simulink model "model1"  (R2019b)
settings: Solver=VariableStepAuto  StartTime=0.0  StopTime=tSimulation  RelTol=1e-3
values from neighbouring files (symbols this model uses):
  a = 1    [param1a.m]    (also in param1b.m = 0.1)
  alpha2 = 3*a    (= 3)    [param1a.m]    (also in param1b.m = 0.3)
  dAmplitude = -1    [param1a.m]    (also in param1b.m)
  Gs = tf(1, den)    [param1a.m]    (also in param1b.m)
  K1 = (alpha1 - a)/b    (= 10)    [param1a.m]    (also in param1b.m = 5; param2.m = 5)
  K2 = alpha2/b    (= 30)    [param1a.m]    (also in param1b.m = 15; param2.m = 2.121)
  tDelay = 0.01    [param1a.m]    (also in param1b.m)
  tDelta = 0.001    [param1a.m]    (also in param1b.m)
  tDist = tSimulation/2    (= 15)    [param1a.m]    (also in param1b.m)
  umax = 999    [param1a.m]    (also in param1b.m = 34)
  umin = -999    [param1a.m]    (also in param1b.m = -10.2)
settings Model: Creator=adityaaaap  LastModifiedBy=adityaaaap

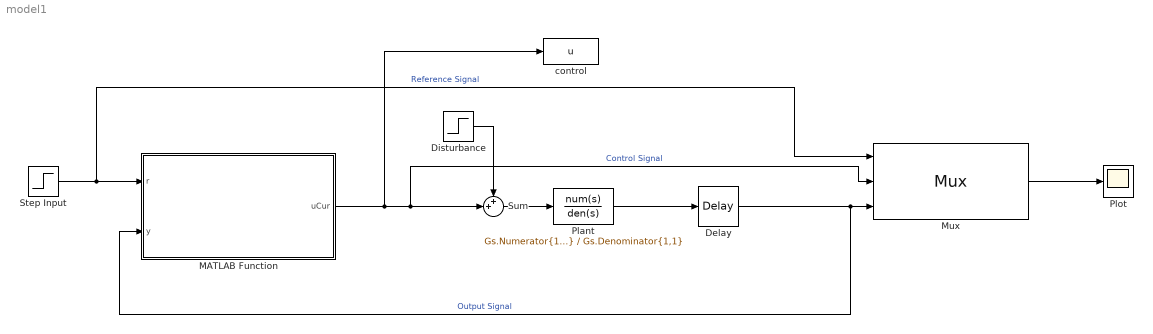
== system model1 ==
  Delay : TransportDelay  DelayTime=tDelay
  Disturbance : Step  Time=tDist  After=dAmplitude  SampleTime=0
  MATLAB Function : MATLAB Function  TreatAsAtomicUnit=on
  Mux : Mux  Inputs=3
      settings: DisplayOption=signals
  Plant : TransferFcn  Numerator=Gs.Numerator{1,1}  Denominator=Gs.Denominator{1,1}
  Plot : Scope
  Step Input : Step  Time=0  SampleTime=tDelta
  Sum : Sum  Inputs=++|
  control : ToWorkspace  VariableName=u
      settings: MaxDataPoints=100000
  wires:
  Plant/1 -> Delay/1
  Sum/1 -> Plant/1
  Disturbance/1 -> Sum/1
  MATLAB Function/1(uCur) -> control/1, Mux/2, Sum/2  "Control Signal"
  Delay/1 -> MATLAB Function/2(y), Mux/3  "Output Signal"
  Mux/1 -> Plot/1
  Step Input/1 -> Mux/1, MATLAB Function/1(r)  "Reference Signal"

== matlab function model1/MATLAB Function ==
  settings: updateMethod=DISCRETE  sampleTime=tDelta
  data: r input; uCur output; y input; K1 parameter; K2 parameter; alpha2 parameter; a parameter; tDelta parameter; umin parameter; umax parameter
function uCur = PIEstim(r,y,K1, K2, alpha2, a, tDelta, umin, umax)
persistent zhat
if isempty(zhat)
    zhat=0;
end
%estimator based MATLAB function with anti-windup
dhat=zhat+K2*(y-r);
uCur= -K1*(y-r)-dhat; 
% if (uCur>umax) uCur=umax;end
% if (uCur<umin) uCur=umin;end
%zhat=zhat-alpha2*zhat*tDelta-tDelta*(y-r)*K2*(alpha2-a)-tDelta*alpha2*udelay(1,ndmax);
zhat=zhat-alpha2*zhat*tDelta-tDelta*(y-r)*K2*(alpha2-a)-tDelta*alpha2*uCur;
